simulink model "BLDCctrlBasedOnMBD"  (R2020b)
settings: Solver=FixedStepDiscrete  StartTime=0.0  StopTime=10.0  FixedStep=0.0001  RelTol=1e-3
PreLoadFcn:
  | load('structMotorCtrl.mat');
  | load('structMBDMotorCrtl.mat');
InitFcn:
  | mbd_s32k_consistency_checks(bdroot(gcs));
undefined symbols (not defined in the file or in its folder): External, LQFP, One, Shot, TRGMUX_PDB_TRIG
libraries: mbd_s32k1xx_ec_toolbox x28, mbd_msd_ec_toolbox x2
settings Model: Creator=k  LastModifiedBy=k
settings DataIOCC: ExternalInput=off  InitialState=off  SaveOutput=off  SignalLogging=off  SaveTime=off
settings OptimizationCC: DefaultParameterBehavior=Inlined  EnhancedBackFolding=on  PassReuseOutputArgsAs=Individual arguments  ZeroExternalMemoryAtStartup=off  ZeroInternalMemoryAtStartup=off  OptimizeBlockOrder=speed  DifferentSizesBufferReuse=on  OptimizationCustomize=off  EfficientTunableParamExpr=on
settings DebuggingCC: InheritedTsInSrcMsg=none  SingleTaskRateTransMsg=error  ParameterTunabilityLossMsg=error  UnconnectedInputMsg=error  UnconnectedOutputMsg=error  UnconnectedLineMsg=error  UnknownTsInhSupMsg=error
settings HardwareCC: ProdBitPerPointer=32  ProdBitPerSizeT=32  ProdBitPerPtrDiffT=32  ProdLargestAtomicInteger=Long  ProdLargestAtomicFloat=Double  ProdWordSize=32  ProdHWDeviceType=ARM Compatible->ARM Cortex
settings ModelReferenceCC: ModelReferenceNumInstancesAllowed=Single
settings SFSimCC: MATLABDynamicMemAlloc=off
settings RTWCC: Description=Model Based Design Toolbox S32K1xx Code Generation Target  SystemTargetFile=mbd_s32k.tlc  MakeCommand=mbd_s32k_make_rtw COPY_MDLREF_INCLUDES=0  TemplateMakefile=mbd_s32k.tmf  GenerateReport=on
settings CodeAppCC: ForceParamTrailComments=on  IgnoreCustomStorageClasses=off  OperatorAnnotations=on  SimulinkDataObjDesc=on  SFDataObjDesc=on  InsertBlockDesc=on
settings STFCustomTargetCC: TargetLangStandard=C99 (ISO)  MultiwordLength=256  ConcurrentExecutionCompliant=off  CombineOutputUpdateFcns=on  ERTCustomFileBanners=on  SupportContinuousTime=off  SupportNonInlinedSFcns=off  RemoveResetFunc=on  MATLABClassNameForMDSCustomization=Simulink.SoftwareTarget.ERTCustomization  CPPClassGenCompliant=off  GRTInterface=off  SystemTargetFile=mbd_s32k.tlc
settings ERTTargetCC: TargetLangStandard=C99 (ISO)  ParMdlRefBuildCompliant=off  CompOptLevelCompliant=off  ConcurrentExecutionCompliant=off  ModelStepFunctionPrototypeControlCompliant=off  CPPClassGenCompliant=off  UseToolchainInfoCompliant=off  InlinedParameterPlacement=NonHierarchical  ERTSrcFileBannerTemplate=mbd_ert_code_template.cgt  ERTHdrFileBannerTemplate=mbd_ert_code_template.cgt  ERTDataSrcFileTemplate=mbd_ert_code_template.cgt  ERTDataHdrFileTemplate=mbd_ert_code_template.cgt  ERTCustomFileTemplate=example_file_process.tlc

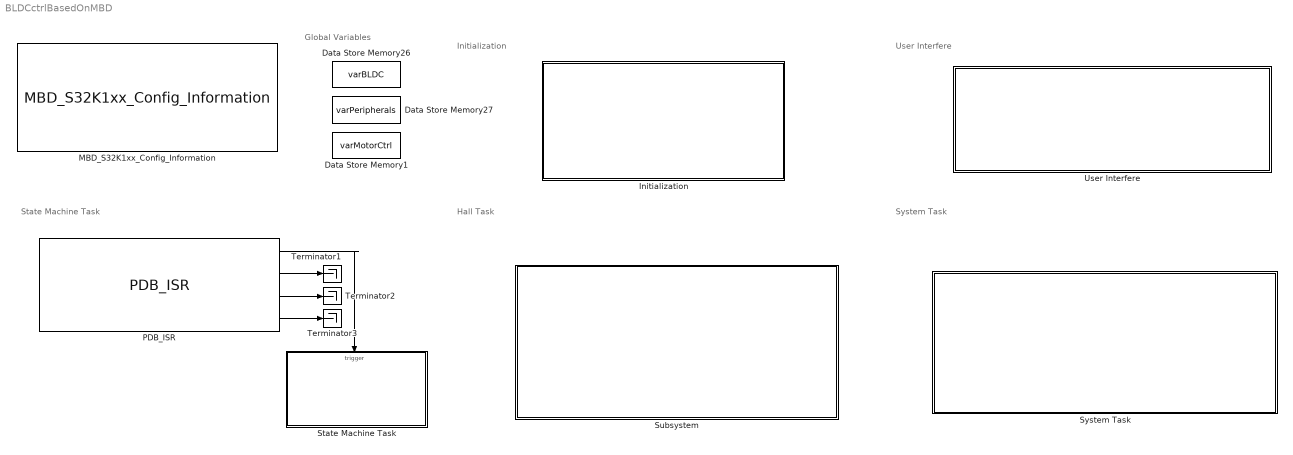
== system BLDCctrlBasedOnMBD ==
  note: State Machine Task
  note: Global Variables
  note: Hall Task
  note: System Task
  note: Initialization
  note: User Interfere
  Data Store Memory1 : DataStoreMemory  DataStoreName=varMotorCtrl  ReadBeforeWriteMsg=warning  WriteAfterWriteMsg=warning  WriteAfterReadMsg=warning  ShowAdditionalParam=off  OutDataTypeStr=Bus: structMotorCtrl
  Data Store Memory26 : DataStoreMemory  DataStoreName=varBLDC  ReadBeforeWriteMsg=warning  WriteAfterWriteMsg=warning  WriteAfterReadMsg=warning  ShowAdditionalParam=off  OutDataTypeStr=Bus: structBLDC
  Data Store Memory27 : DataStoreMemory  DataStoreName=varPeripherals  ReadBeforeWriteMsg=warning  WriteAfterWriteMsg=warning  WriteAfterReadMsg=warning  ShowAdditionalParam=off  OutDataTypeStr=Bus: structPeripherals
  Initialization : Subsystem
  MBD_S32K1xx_Config_Information : mbd_s32k1xx_ec_toolbox/MBD_S32K1xx_Config_Information  mbdt_ver=0  disp_str=|  config_params=[]  mcu_target_name=S32K144  mcu_target_package=100-LQFP  mcu_target_sram_size=64KB  mcu_system_clock_freq=80  mcu_xtal_freq=External 8  mcu_steptick_timer=LPIT Channel 0  mcu_steptick_prio=15  ds_import_enable=on  target_compiler=GCC  target_memory=FLASH  gcc_target_compile_opts=-mthumb -mfloat-abi=hard -mfpu=fpv4-sp-d16 -O1 -g -gstrict-dwarf  gcc_target_assemble_opts=-mthumb -mfloat-abi=hard -mfpu=fpv4-sp-d16 -g  gcc_target_link_opts=-mthumb -mfloat-abi=hard -mfpu=fpv4-sp-d16  gcc_target_default_lcf=on  gcc_target_user_lcf=S32K148_192_flash.ld  ghs_target_compile_opts=-cpu=cortexm4f -thumb -fpu=vfpv4_d16 -fsingle -Ogeneral -Wundef -Wimplicit-int -Wshadow -Wtrigraphs --no_commons --gnu_asm -gnu99 -gdwarf-2 -G  ghs_target_assemble_opts=-cpu=cortexm4f -fpu=vfpv4_d16  ghs_target_link_opts=-cpu=cortexm4f -thumb -fpu=vfpv4_d16  ghs_target_default_lcf=on  ghs_target_user_lcf=S32K148_192_flash.ld  iar_target_compile_opts=--cpu=Cortex-M4F --thumb --fpu=VFPv4_sp -Ol -e --debug --dlib_config normal  iar_target_assemble_opts=--cpu Cortex-M4F --thumb --fpu VFPv4_sp  iar_target_link_opts=--no_exceptions --vfe --inline  iar_target_default_lcf=on  iar_target_user_lcf=S32K148_192_flash.icf  pil_download_enable=off  rbl_download_enable=on  rbl_start_delay=5000  rbl_download_interface=OpenSDA  rbl_restart_request=off  rbl_com_port=Custom  rbl_com_port_custom=COM1  pil_download_rate=57600  pil_opensda_drive=Custom  pil_opensda_drive_custom=E  pil_uart_instance=1  pil_uart_rx=PTC6: [LPUART1_RX | Receive]  pil_uart_tx=PTC7: [LPUART1_TX | Transmit]  FTM_PWM_PcrCheckEnDis=on  FTM_Input_Edge_Inputs_PcrCheckEnDis=on  FTM_Dual_Edge_Inputs_PcrCheckEnDis=on  FTM_Quadrature_Inputs_PcrCheckEnDis=on  FTM_Hall_Sensor_Inputs_PcrCheckEnDis=on  LPTMR_PcrCheckEnDis=on  PIT_PcrCheckEnDis=on  RTC_PcrCheckEnDis=on  FlexCAN_PcrCheckEnDis=on  LIN_PcrCheckEnDis=on  FlexIO_PcrCheckEnDis=on  LPI2C_PcrCheckEnDis=on  LPSPI_PcrCheckEnDis=on  LPUART_PcrCheckEnDis=on  CMP_PcrCheckEnDis=on  GPIO_OutputPcrCheckEnDis=on  GPIO_InputPcrCheckEnDis=on  SBC_PcrCheckEnDis=on  BMS_PcrCheckEnDis=on  AMMCLIB_PcrCheckEnDis=on  FM_PcrCheckEnDis=on  Profile_PcrCheckEnDis=on  ConfigParams_PcrCheckEnDis=on  ModelRef_PcrCheckEnDis=on  PDB0_PcrCheckEnDis=on  CSEc_PcrCheckEnDis=on  eDMA_PcrCheckEnDis=on  FLASH_PcrCheckEnDis=on  ADC_PcrCheckEnDis=on  WDOG_PcrCheckEnDis=on
      | Target : S32K144-64KB_SRAM
      | Package : 100-pin
      | System clock : 80 MHz
      | XTAL clock : External 8 MHz
      | Compiler : IAR
      | Target Type : FLASH
      | Download Code after build : off
      | Step Tick Interrupt Priority : 15
  PDB_ISR : mbd_s32k1xx_ec_toolbox/Motor Control Blocks/PDB Blocks/PDB_ISR  Priority=2  pdbModule=0  prioInterrupt=10  regScPdbie=on  regScPdbeie=off  regIdlyIdly=2000
  State Machine Task : Subsystem
  Subsystem : Subsystem
  System Task : Subsystem
  Terminator1 : Terminator
  Terminator2 : Terminator
  Terminator3 : Terminator
  User Interfere : Subsystem
  wires:
  PDB_ISR/2 -> Terminator1/1
  PDB_ISR/3 -> Terminator2/1
  PDB_ISR/4 -> Terminator3/1
  PDB_ISR/1 -> State Machine Task/Trigger

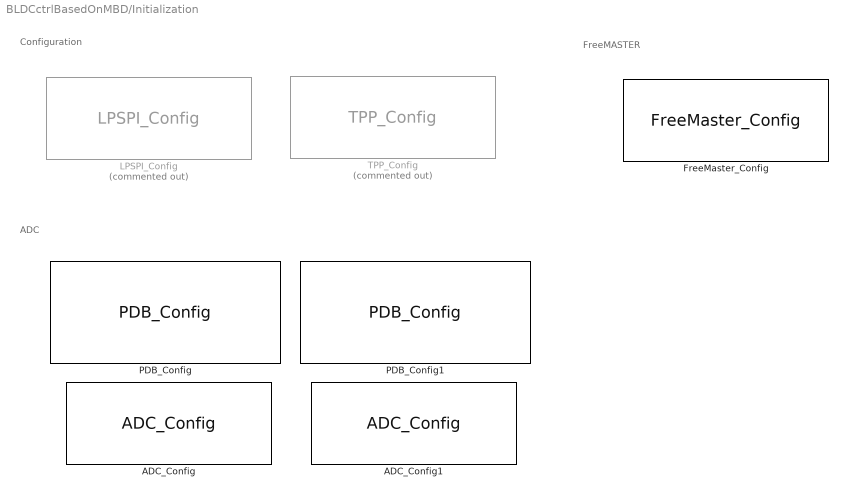
== system BLDCctrlBasedOnMBD/Initialization ==
  note: FreeMASTER
  note: ADC
  note: Configuration
  ADC_Config : mbd_s32k1xx_ec_toolbox/Motor Control Blocks/ADC Blocks/ADC_Config  instance=0  mode=12-bit conversion  smplts=20  adiclk=alternate clock 1  adiv=input clock  show_adv_opts=on  pretrgsel=PDB pre-trigger  swpretrg=Disabled  adtrg=hardware  trgsel=PDB output  refsel=Vrefh and Vrefl  supply_monitoring=off  acfe=off  acfgt=off  acren=off  cv1=0  cv2=0  adco=off  avge=off  avgs=4 samples
  ADC_Config1 : mbd_s32k1xx_ec_toolbox/Motor Control Blocks/ADC Blocks/ADC_Config  instance=1  mode=12-bit conversion  smplts=20  adiclk=alternate clock 1  adiv=input clock  show_adv_opts=on  pretrgsel=PDB pre-trigger  swpretrg=Disabled  adtrg=hardware  trgsel=PDB output  refsel=Vrefh and Vrefl  supply_monitoring=off  acfe=off  acfgt=off  acren=off  cv1=0  cv2=0  adco=off  avge=off  avgs=4 samples
  FreeMaster_Config : mbd_s32k1xx_ec_toolbox/Utility Blocks/FreeMaster_Config  interface=LPUART1  baudrate=115200  rxd=PTC6: [LPUART1_RX | Receive]  txd=PTC7: [LPUART1_TX | Transmit]  mode=Poll-driven  isr_prio=15  show_adv_opts=on  use_scope=on  max_scope_vars=8  use_recorder=on  max_rec_vars=8  rec_buff_size=1024  rec_timebase=0 seconds  comm_buffer_size_auto=on  comm_buffer_size=255  comm_rqueue_size_default=on  comm_rqueue_size=32
  "LPSPI_Config " : mbd_s32k1xx_ec_toolbox/Communication Blocks/SPI Blocks/LPSPI_Config   Commented=on  InstanceNumber=0  Role=Master  BaudRate=2000000  ShowAdvanced=on  sin=PTB3: [LPSPI0_SIN | LPSPI Serial Data Input]  sout=PTB4: [LPSPI0_SOUT | LPSPI Serial Data Output]  sck=PTB2: [LPSPI0_SCK | LPSPI Serial Clock I/O]  pcs0=None  pcs1=None  pcs2=None  pcs3=None  CPHA=1  CPOL=0  BitOrder=MSB first  TransferSize=8  WhichPCS=0  PCSPol=ActiveLow  ContinuousTransfer=off
  PDB_Config : mbd_s32k1xx_ec_toolbox/Motor Control Blocks/PDB Blocks/PDB_Config  pdbModule=0  regScCont=One-Shot  regScTrgsel=External (TRGMUX_PDB_TRIG)  trgMuxSel=FTM3 Initialize Trigger  trgMuxSelPin=PTB5: [TRGMUX_IN0 | Trigger Mux Input]  regModModulus=3900  regScPrescaler=1  regScMult=1  regPoenPoen0=off  regPo0DlyDly1=0  regPo0DlyDly2=0  enable_pdb_init=on  show_adv_opts=on  regCh0C1En0=on  regCh0C1En1=on  regCh0C1En2=on  regCh0C1En3=on  regCh0C1En4=off  regCh0C1En5=off  regCh0C1En6=off  regCh0C1En7=off  regCh0C1Bb0=off  regCh0C1Bb1=off  regCh0C1Bb2=off  regCh0C1Bb3=off  regCh0C1Bb4=off  regCh0C1Bb5=off  regCh0C1Bb6=off  regCh0C1Bb7=off  regCh0C1Tos0=Pre-trigger is in delay mode  regCh0C1Tos1=Pre-trigger is in delay mode  regCh0C1Tos2=Pre-trigger is in delay mode  regCh0C1Tos3=Pre-trigger is in delay mode  regCh0C1Tos4=Pre-trigger is in delay mode  regCh0C1Tos5=Pre-trigger is in delay mode  regCh0C1Tos6=Pre-trigger is in delay mode  regCh0C1Tos7=Pre-trigger is in delay mode  regCh0DlyDly0=0  regCh0DlyDly1=500  regCh0DlyDly2=1000  regCh0DlyDly3=1500  regCh0DlyDly4=0  regCh0DlyDly5=0  regCh0DlyDly6=0  regCh0DlyDly7=0  regCh1C1En0=off  regCh1C1En1=off  regCh1C1En2=off  regCh1C1En3=off  regCh1C1En4=off  regCh1C1En5=off  regCh1C1En6=off  regCh1C1En7=off  regCh1C1Bb0=off  regCh1C1Bb1=off  regCh1C1Bb2=off  regCh1C1Bb3=off  regCh1C1Bb4=off  regCh1C1Bb5=off  regCh1C1Bb6=off  regCh1C1Bb7=off  regCh1C1Tos0=Pre-trigger is in delay mode  regCh1C1Tos1=Pre-trigger is in delay mode  regCh1C1Tos2=Pre-trigger is in delay mode  regCh1C1Tos3=Pre-trigger is in delay mode  regCh1C1Tos4=Pre-trigger is in delay mode  regCh1C1Tos5=Pre-trigger is in delay mode  regCh1C1Tos6=Pre-trigger is in delay mode  regCh1C1Tos7=Pre-trigger is in delay mode  regCh1DlyDly0=0  regCh1DlyDly1=0  regCh1DlyDly2=0  regCh1DlyDly3=0  regCh1DlyDly4=0  regCh1DlyDly5=0  regCh1DlyDly6=0  regCh1DlyDly7=0
  PDB_Config1 : mbd_s32k1xx_ec_toolbox/Motor Control Blocks/PDB Blocks/PDB_Config  pdbModule=1  regScCont=One-Shot  regScTrgsel=External (TRGMUX_PDB_TRIG)  trgMuxSel=FTM3 Initialize Trigger  trgMuxSelPin=PTB5: [TRGMUX_IN0 | Trigger Mux Input]  regModModulus=3900  regScPrescaler=1  regScMult=1  regPoenPoen0=off  regPo0DlyDly1=0  regPo0DlyDly2=0  enable_pdb_init=on  show_adv_opts=on  regCh0C1En0=on  regCh0C1En1=on  regCh0C1En2=off  regCh0C1En3=off  regCh0C1En4=off  regCh0C1En5=off  regCh0C1En6=off  regCh0C1En7=off  regCh0C1Bb0=off  regCh0C1Bb1=off  regCh0C1Bb2=off  regCh0C1Bb3=off  regCh0C1Bb4=off  regCh0C1Bb5=off  regCh0C1Bb6=off  regCh0C1Bb7=off  regCh0C1Tos0=Pre-trigger is in delay mode  regCh0C1Tos1=Pre-trigger is in delay mode  regCh0C1Tos2=Pre-trigger is in delay mode  regCh0C1Tos3=Pre-trigger is in delay mode  regCh0C1Tos4=Pre-trigger is in delay mode  regCh0C1Tos5=Pre-trigger is in delay mode  regCh0C1Tos6=Pre-trigger is in delay mode  regCh0C1Tos7=Pre-trigger is in delay mode  regCh0DlyDly0=0  regCh0DlyDly1=1000  regCh0DlyDly2=0  regCh0DlyDly3=0  regCh0DlyDly4=0  regCh0DlyDly5=0  regCh0DlyDly6=0  regCh0DlyDly7=0  regCh1C1En0=off  regCh1C1En1=off  regCh1C1En2=off  regCh1C1En3=off  regCh1C1En4=off  regCh1C1En5=off  regCh1C1En6=off  regCh1C1En7=off  regCh1C1Bb0=off  regCh1C1Bb1=off  regCh1C1Bb2=off  regCh1C1Bb3=off  regCh1C1Bb4=off  regCh1C1Bb5=off  regCh1C1Bb6=off  regCh1C1Bb7=off  regCh1C1Tos0=Pre-trigger is in delay mode  regCh1C1Tos1=Pre-trigger is in delay mode  regCh1C1Tos2=Pre-trigger is in delay mode  regCh1C1Tos3=Pre-trigger is in delay mode  regCh1C1Tos4=Pre-trigger is in delay mode  regCh1C1Tos5=Pre-trigger is in delay mode  regCh1C1Tos6=Pre-trigger is in delay mode  regCh1C1Tos7=Pre-trigger is in delay mode  regCh1DlyDly0=0  regCh1DlyDly1=0  regCh1DlyDly2=0  regCh1DlyDly3=0  regCh1DlyDly4=0  regCh1DlyDly5=0  regCh1DlyDly6=0  regCh1DlyDly7=0
  TPP_Config : mbd_msd_ec_toolbox/TPP/TPP_Config  Priority=1  Commented=on  tppInstance=0  desatMode=off  fullonMode=on  lockMode=off  overtempEvent=on  phaseEvent=on  desatEvent=on  framingEvent=on  vlsEvent=on  writeErrEvent=on  overcurrentEvent=on  resetEvent=on  mcuTppIntEn=on  prioInt=15  tppDeadtime=500  initTppNow=on  tppSpiInst=Please add SPI block to workspace  tppPwmModule=Please add FTM block to workspace  tppPair0_1=on  tppPair2_3=on  tppPair4_5=on  tppPair6_7=off  tppFirstChHS=on  tppEn1Pin=PTA2: [PTA2 | Port A I/O]  tppEn2Pin=PTA2: [PTA2 | Port A I/O]  tppRstPin=PTA3: [PTA3 | Port A I/O]  tppCsPin=PTB5: [PTB5 | Port B I/O]  tppIntPin=PTE10: [PTE10 | Port E I/O]

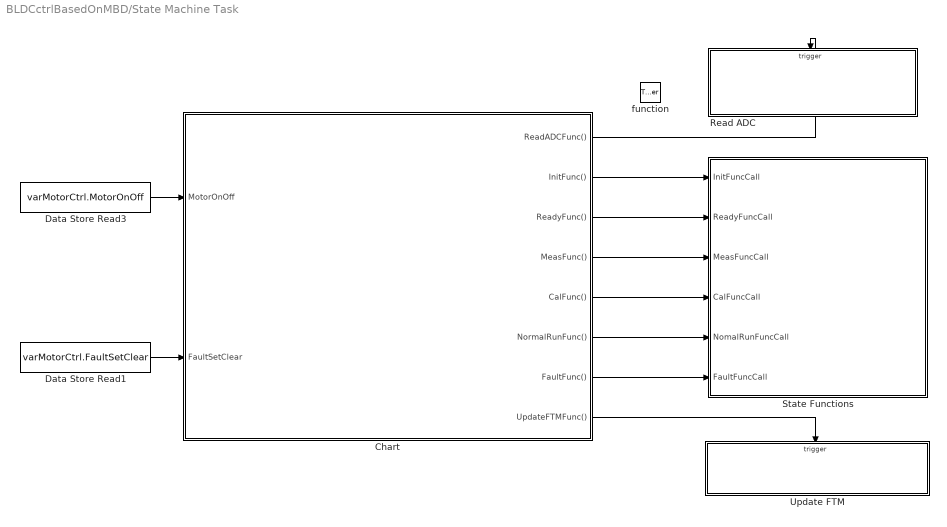
== system BLDCctrlBasedOnMBD/State Machine Task ==
  function : TriggerPort  TriggerType=function-call  VariantControl=Variant
  Chart : Stateflow chart  TreatAsAtomicUnit=on
      settings: PortSchema="{\"entries\":[{\"content\":{\"sides\":[{\"content\":{\"connectorIds\":[\"In1\",\"In2\"]},\"type\":\"ConnectorPlacement.EquallySpacedRectSide\",\"uuid\":\"6aab3670-dbd5-4778-9051-de706f320d6c\"},{\"content\":{\"connectorIds\":[\"Out7\",\"Out2\",\"Out3\",\"Out1\",\"Out4\",\"Out5\",\"Out6\",\"Out8\"],\"side\":\"RIGHT\"},\"type\":\"ConnectorPlacement.EquallySpacedRectSide\",\"uuid\":\"2f9f0170-7a01-4f36-b182-da63b20b6c86\"},{\"content\":{\"connectorIds\":[],\"side\":\"TOP\"},\"type\":\"ConnectorPlacement.EquallySpacedRectSide\",\"uuid\":\"ed2088fa-8282-455e-b501-bc381afe58e4\"},{\"content\":{\"connectorIds\":[],\"side\":\"HIDDEN\"},\"type\":\"ConnectorPlacement.EquallySpacedRectSide\",\"uuid\":\"d652818b-6052-4db5-9e3c-1b8d8b3f5bf8\"}]},\"type\":\"ConnectorPlacement.EquallySpacedConnector\",\"uuid\":\"e57e4f41-1290-4580-a9fc-0c62073a8c32\"}],\"packageUris\":[\"http://schema.mathworks.com/mf0/Connector/R2020b\"],\"version\":\"1.0\"}"
  Data Store Read1 : DataStoreRead  DataStoreName=varMotorCtrl  DataStoreElements=varMotorCtrl.FaultSetClear
  Data Store Read3 : DataStoreRead  DataStoreName=varMotorCtrl  DataStoreElements=varMotorCtrl.MotorOnOff
  Read ADC : Subsystem  TreatAsAtomicUnit=on
  State Functions : Subsystem  Priority=1
  Update FTM : Subsystem
  wires:
  Data Store Read3/1 -> Chart/1(MotorOnOff)
  Data Store Read1/1 -> Chart/2(FaultSetClear)
  Chart/7(ReadADCFunc()) -> Read ADC/Trigger
  Chart/8(UpdateFTMFunc()) -> Update FTM/Trigger
  Chart/2(InitFunc()) -> State Functions/1(InitFuncCall)
  Chart/3(ReadyFunc()) -> State Functions/2(ReadyFuncCall)
  Chart/1(MeasFunc()) -> State Functions/3(MeasFuncCall)
  Chart/4(CalFunc()) -> State Functions/4(CalFuncCall)
  Chart/5(NormalRunFunc()) -> State Functions/5(NomalRunFuncCall)
  Chart/6(FaultFunc()) -> State Functions/6(FaultFuncCall)

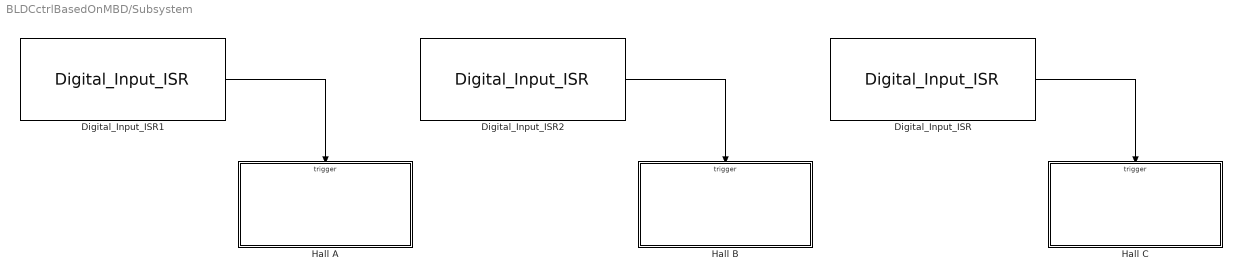
== system BLDCctrlBasedOnMBD/Subsystem ==
  Digital_Input_ISR : mbd_s32k1xx_ec_toolbox/GPIO Blocks/Digital_Input_ISR  gpio_pin=PTA1: [PTA1 | Port A I/O]  irqc=on either-edge  prio=5
  Digital_Input_ISR1 : mbd_s32k1xx_ec_toolbox/GPIO Blocks/Digital_Input_ISR  gpio_pin=PTA15: [PTA15 | Port A I/O]  irqc=on either-edge  prio=5
  Digital_Input_ISR2 : mbd_s32k1xx_ec_toolbox/GPIO Blocks/Digital_Input_ISR  gpio_pin=PTA16: [PTA16 | Port A I/O]  irqc=on either-edge  prio=5
  Hall A : Subsystem  TreatAsAtomicUnit=on
  Hall B : Subsystem  TreatAsAtomicUnit=on
  Hall C : Subsystem  TreatAsAtomicUnit=on
  wires:
  Digital_Input_ISR/1 -> Hall C/Trigger
  Digital_Input_ISR1/1 -> Hall A/Trigger
  Digital_Input_ISR2/1 -> Hall B/Trigger

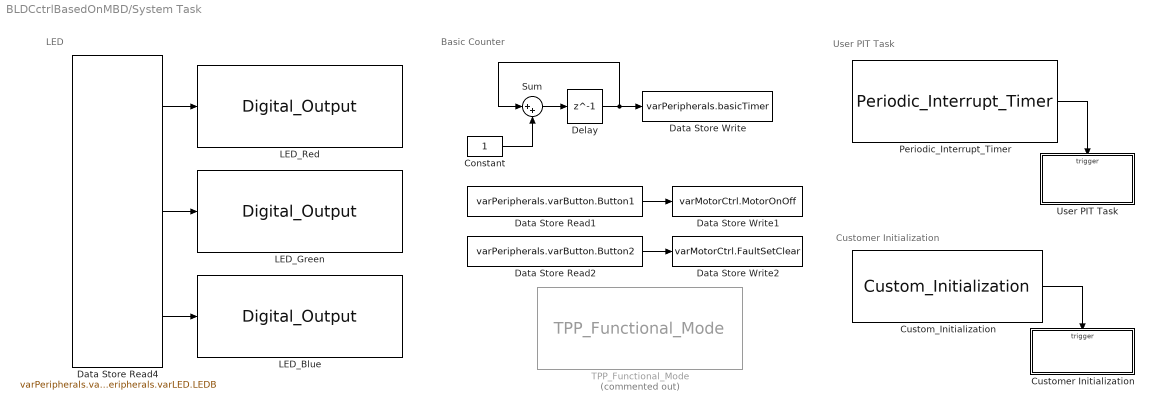
== system BLDCctrlBasedOnMBD/System Task ==
  note: LED
  note: Basic Counter
  note: User PIT Task
  note: Customer Initialization
  Constant : Constant  OutDataTypeStr=uint32
  Custom_Initialization : mbd_s32k1xx_ec_toolbox/Utility Blocks/Custom_Initialization
  Customer Initialization : Subsystem  TreatAsAtomicUnit=on
  Data Store Read1 : DataStoreRead  DataStoreName=varPeripherals  DataStoreElements=varPeripherals.varButton.Button1
  Data Store Read2 : DataStoreRead  DataStoreName=varPeripherals  DataStoreElements=varPeripherals.varButton.Button2
  Data Store Read4 : DataStoreRead  DataStoreName=varPeripherals  DataStoreElements=varPeripherals.varLED.LEDR#varPeripherals.varLED.LEDG#varPeripherals.varLED.LEDB
  Data Store Write : DataStoreWrite  DataStoreName=varPeripherals  DataStoreElements=varPeripherals.basicTimer
  Data Store Write1 : DataStoreWrite  DataStoreName=varMotorCtrl  DataStoreElements=varMotorCtrl.MotorOnOff
  Data Store Write2 : DataStoreWrite  DataStoreName=varMotorCtrl  DataStoreElements=varMotorCtrl.FaultSetClear
  Delay : Delay  DelayLength=1  InitialCondition=0
  LED_Blue : mbd_s32k1xx_ec_toolbox/GPIO Blocks/Digital_Output  gpio_pin=PTD0: [PTD0 | Port D I/O]  init_val=High  drive_strength=Low
  LED_Green : mbd_s32k1xx_ec_toolbox/GPIO Blocks/Digital_Output  gpio_pin=PTD16: [PTD16 | Port D I/O]  init_val=High  drive_strength=Low
  LED_Red : mbd_s32k1xx_ec_toolbox/GPIO Blocks/Digital_Output  gpio_pin=PTD15: [PTD15 | Port D I/O]  init_val=High  drive_strength=Low
  Periodic_Interrupt_Timer : mbd_s32k1xx_ec_toolbox/Utility Blocks/Periodic_Interrupt_Timer  channel=1  period=500000  prio=14  startCounter=on
  Sum : Sum  Inputs=|++
  TPP_Functional_Mode : mbd_msd_ec_toolbox/TPP/TPP_Functional_Mode  Commented=on  tppInstance=0  action=Sleep
  User PIT Task : Subsystem  TreatAsAtomicUnit=on
  wires:
  Data Store Read4/1 -> LED_Red/1
  Data Store Read4/2 -> LED_Green/1
  Data Store Read4/3 -> LED_Blue/1
  Constant/1 -> Sum/2
  Delay/1 -> Data Store Write/1, Sum/1
  Sum/1 -> Delay/1
  Periodic_Interrupt_Timer/1 -> User PIT Task/Trigger
  Custom_Initialization/1 -> Customer Initialization/Trigger
  Data Store Read1/1 -> Data Store Write1/1
  Data Store Read2/1 -> Data Store Write2/1

== system BLDCctrlBasedOnMBD/User Interfere ==
  note: User Button
  Digital_Input_ISR : mbd_s32k1xx_ec_toolbox/GPIO Blocks/Digital_Input_ISR  gpio_pin=PTC12: [PTC12 | Port C I/O]  irqc=on rising-edge  prio=13
  Digital_Input_ISR1 : mbd_s32k1xx_ec_toolbox/GPIO Blocks/Digital_Input_ISR  gpio_pin=PTC13: [PTC13 | Port C I/O]  irqc=on rising-edge  prio=13
  Function-Call Subsystem1 : Subsystem  TreatAsAtomicUnit=on
  Function-Call Subsystem2 : Subsystem  TreatAsAtomicUnit=on
  wires:
  Digital_Input_ISR/1 -> Function-Call Subsystem2/Trigger
  Digital_Input_ISR1/1 -> Function-Call Subsystem1/Trigger

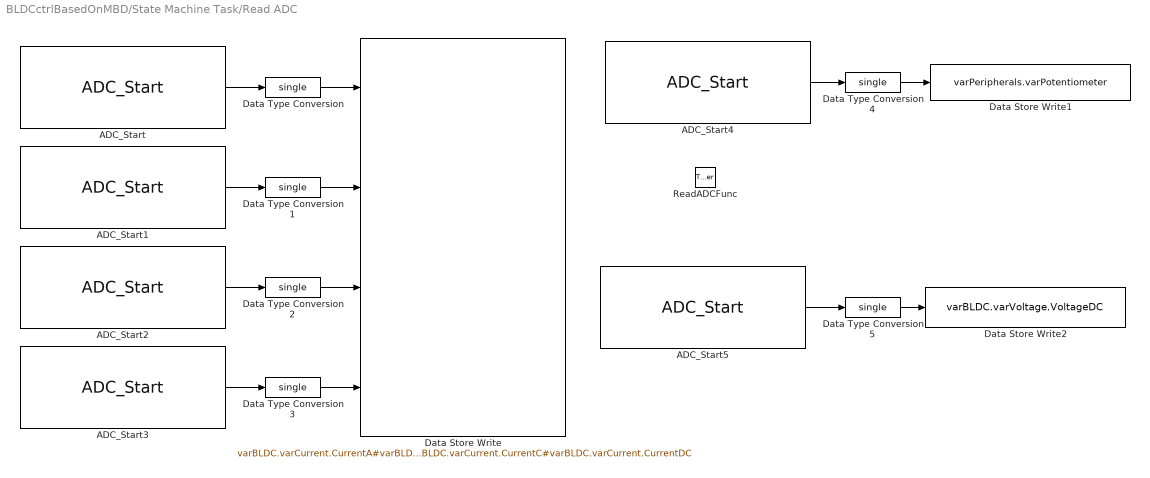
== system BLDCctrlBasedOnMBD/State Machine Task/Read ADC ==
  ReadADCFunc : TriggerPort  TriggerType=function-call  VariantControl=Variant
  ADC_Start : mbd_s32k1xx_ec_toolbox/Motor Control Blocks/ADC Blocks/ADC_Start  instance=0  adc_r=A  adc_chan=VREFSH  aien=off  mcuTargetUpdate=on
  ADC_Start1 : mbd_s32k1xx_ec_toolbox/Motor Control Blocks/ADC Blocks/ADC_Start  instance=0  adc_r=B  adc_chan=VREFSL  aien=off  mcuTargetUpdate=on
  ADC_Start2 : mbd_s32k1xx_ec_toolbox/Motor Control Blocks/ADC Blocks/ADC_Start  instance=0  adc_r=C  adc_chan=VDD 3V  aien=off  mcuTargetUpdate=on
  ADC_Start3 : mbd_s32k1xx_ec_toolbox/Motor Control Blocks/ADC Blocks/ADC_Start  instance=0  adc_r=D  adc_chan=PTC14: [ADC0_SE12 | ADC Single Ended Input]  aien=off  mcuTargetUpdate=on
  ADC_Start4 : mbd_s32k1xx_ec_toolbox/Motor Control Blocks/ADC Blocks/ADC_Start  instance=1  adc_r=A  adc_chan=VREFSH  aien=off  mcuTargetUpdate=on
  ADC_Start5 : mbd_s32k1xx_ec_toolbox/Motor Control Blocks/ADC Blocks/ADC_Start  instance=1  adc_r=B  adc_chan=VREFSL  aien=off  mcuTargetUpdate=on
  Data Store Write : DataStoreWrite  DataStoreName=varBLDC  DataStoreElements=varBLDC.varCurrent.CurrentA#varBLDC.varCurrent.CurrentB#varBLDC.varCurrent.CurrentC#varBLDC.varCurrent.CurrentDC
  Data Store Write1 : DataStoreWrite  DataStoreName=varPeripherals  DataStoreElements=varPeripherals.varPotentiometer
  Data Store Write2 : DataStoreWrite  DataStoreName=varBLDC  DataStoreElements=varBLDC.varVoltage.VoltageDC
  Data Type Conversion{,1..5} (6 alike) : DataTypeConversion  OutDataTypeStr=single
  wires:
  ADC_Start/1 -> Data Type Conversion/1
  ADC_Start1/1 -> Data Type Conversion1/1
  ADC_Start2/1 -> Data Type Conversion2/1
  ADC_Start3/1 -> Data Type Conversion3/1
  ADC_Start4/1 -> Data Type Conversion4/1
  ADC_Start5/1 -> Data Type Conversion5/1
  Data Type Conversion/1 -> Data Store Write/1
  Data Type Conversion1/1 -> Data Store Write/2
  Data Type Conversion2/1 -> Data Store Write/3
  Data Type Conversion3/1 -> Data Store Write/4
  Data Type Conversion4/1 -> Data Store Write1/1
  Data Type Conversion5/1 -> Data Store Write2/1

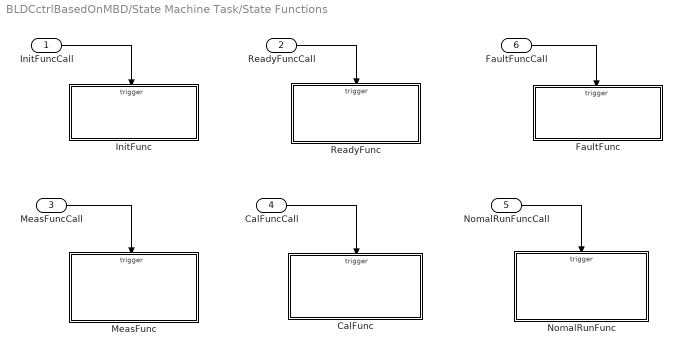
== system BLDCctrlBasedOnMBD/State Machine Task/State Functions ==
  InitFuncCall : Inport
  ReadyFuncCall : Inport  Port=2
  MeasFuncCall : Inport  Port=3
  CalFuncCall : Inport  Port=4
  NomalRunFuncCall : Inport  Port=5
  FaultFuncCall : Inport  Port=6
  CalFunc : Subsystem  TreatAsAtomicUnit=on
  FaultFunc : Subsystem  TreatAsAtomicUnit=on
  InitFunc : Subsystem  TreatAsAtomicUnit=on
  MeasFunc : Subsystem  TreatAsAtomicUnit=on
  NomalRunFunc : Subsystem  TreatAsAtomicUnit=on
  ReadyFunc : Subsystem  TreatAsAtomicUnit=on
  wires:
  MeasFuncCall/1 -> MeasFunc/Trigger
  CalFuncCall/1 -> CalFunc/Trigger
  InitFuncCall/1 -> InitFunc/Trigger
  ReadyFuncCall/1 -> ReadyFunc/Trigger
  FaultFuncCall/1 -> FaultFunc/Trigger
  NomalRunFuncCall/1 -> NomalRunFunc/Trigger

== system BLDCctrlBasedOnMBD/State Machine Task/Update FTM ==
  UpdateFTMFunc : TriggerPort  TriggerType=function-call  VariantControl=Variant
  Data Store Read2 : DataStoreRead  DataStoreName=varBLDC  DataStoreElements=varBLDC.varDuty.DutyA#varBLDC.varDuty.DutyB#varBLDC.varDuty.DutyC
  FTM_PWM_Config : mbd_s32k1xx_ec_toolbox/Motor Control Blocks/FTM Blocks/FTM_PWM_Config  Priority=5  ftmModule=3  ftmMode=Center-Aligned PWM  ftmSourceClock=80 MHz  swcontrol_enable=off  chan0En=on  chan0Type=Independent  chan2En=on  chan2Type=Independent  chan4En=on  chan4Type=Independent  chan6En=off  chan6Type=Independent  ftmPwmUnits=Hz  outFrequency=20000  ftmPeriod=4000  ftmPrescaler=Divide by 1  deadtimeUnits=Nanoseconds  deadtimeNs=0  deadtimeTicks=0  deadtimePrescaler=Divide by 1  dutyCycleCh0=0  dutyCycleCh1=0  dutyCycleCh2=0  dutyCycleCh3=0  dutyCycleCh4=0  dutyCycleCh5=0  dutyCycleCh6=0.25  dutyCycleCh7=0.25  dutyCycleSim=off  startAfterInit=on  showAdvOpt=on  pinFtmCh0=PTB8: [FTM3_CH0 | FTM Channel]  pinFtmCh1=PTB9: [FTM3_CH1 | FTM Channel]  pinPolCh0=Active Low  pinPolCh1=Active High  outputComplem0=Main duplicated  outputLevel0=Low  outputLevel1=Low  pinFtmCh2=PTB10: [FTM3_CH2 | FTM Channel]  pinFtmCh3=PTB11: [FTM3_CH3 | FTM Channel]  pinPolCh2=Active Low  pinPolCh3=Active High  outputComplem2=Main duplicated  outputLevel2=Low  outputLevel3=Low  pinFtmCh4=PTC10: [FTM3_CH4 | FTM Channel]  pinFtmCh5=PTC11: [FTM3_CH5 | FTM Channel]  pinPolCh4=Active Low  pinPolCh5=Active High  outputComplem4=Main duplicated  outputLevel4=Low  outputLevel5=Low  pinFtmCh6=PTC12: [FTM3_CH6 | FTM Channel]  pinFtmCh7=None  pinPolCh6=Active Low  pinPolCh7=Active Low  outputComplem6=Main duplicated  outputLevel6=Low  outputLevel7=Low  initTrigger=on  chTrigger0=off  chTrigger1=off  chTrigger2=off  chTrigger3=off  chTrigger4=off  chTrigger5=off  chTrigger6=off  chTrigger7=off  mcuTargetUpdate=on  pwmSyncTrg=Software trigger  pwmSyncHwRouting=TRGMUX_FTM7  pwmSyncTrg0=off  pwmSyncTrg1=off  pwmSyncTrg2=off  pwmSyncAutoClear=off  pwmSyncMinLoad=on  pwmSyncMaxLoad=off  pwmSyncInvert=PWM Syncronization  pwmSyncOutControl=PWM Syncronization  pwmSyncOutMask=PWM Syncronization  pwmSyncCounterInitial=PWM Syncronization  pwmSyncPoints=Wait Loading Points  reloadEnable=off  reloadPriority=15  reloadHalfCycle=off  reloadHCR=0  reloadFrequency=0  chnMatch0=off  chnMatch1=off  chnMatch2=off  chnMatch3=off  chnMatch4=off  chnMatch5=off  chnMatch6=off  chnMatch7=off  pwmFaultProtection=off  pwmFaultInterrupt=off  pwmFaultClearing=Fault control disabled  pwmFaultPinState=Safe Value  pwmFaultFilterValue=0  pwmFaultPriority=15  fault_disen_0=off  fault_filter_0=off  fault_polarity_0=Active High  fault_disen_1=off  fault_filter_1=off  fault_polarity_1=Active high  fault_disen_2=off  fault_filter_2=off  fault_polarity_2=Active high  fault_disen_3=off  fault_filter_3=off  fault_polarity_3=Active high  fault_pin_0=None  fault_pin_1=None  fault_pin_2=None  fault_pin_3=None
  wires:
  Data Store Read2/1 -> FTM_PWM_Config/1, FTM_PWM_Config/2
  Data Store Read2/3 -> FTM_PWM_Config/5, FTM_PWM_Config/6
  Data Store Read2/2 -> FTM_PWM_Config/3, FTM_PWM_Config/4

== system BLDCctrlBasedOnMBD/Subsystem/Hall A ==
  ReadHallA : TriggerPort  TriggerType=function-call  VariantControl=Variant
  Data Store Write1 : DataStoreWrite  DataStoreName=varBLDC  DataStoreElements=varBLDC.varHall.HallA
  Digital_Input_HALL_A : mbd_s32k1xx_ec_toolbox/GPIO Blocks/Digital_Input  gpio_pin=PTA15: [PTA15 | Port A I/O]  pull_resistor=None  passive_filter=off
  wires:
  Digital_Input_HALL_A/1 -> Data Store Write1/1

== system BLDCctrlBasedOnMBD/Subsystem/Hall B ==
  ReadHallA : TriggerPort  TriggerType=function-call  VariantControl=Variant
  Data Store Write1 : DataStoreWrite  DataStoreName=varBLDC  DataStoreElements=varBLDC.varHall.HallB
  Digital_Input_HALL_B : mbd_s32k1xx_ec_toolbox/GPIO Blocks/Digital_Input  gpio_pin=PTA16: [PTA16 | Port A I/O]  pull_resistor=None  passive_filter=off
  wires:
  Digital_Input_HALL_B/1 -> Data Store Write1/1

== system BLDCctrlBasedOnMBD/Subsystem/Hall C ==
  ReadHallA : TriggerPort  TriggerType=function-call  VariantControl=Variant
  Data Store Write1 : DataStoreWrite  DataStoreName=varBLDC  DataStoreElements=varBLDC.varHall.HallC
  Digital_Input_HALL_C : mbd_s32k1xx_ec_toolbox/GPIO Blocks/Digital_Input  gpio_pin=PTA1: [PTA1 | Port A I/O]  pull_resistor=None  passive_filter=off
  wires:
  Digital_Input_HALL_C/1 -> Data Store Write1/1

== system BLDCctrlBasedOnMBD/System Task/Customer Initialization ==
  CustInit : TriggerPort  TriggerType=function-call  VariantControl=Variant
  0_uint32 : Constant  Value=0  OutDataTypeStr=uint32
  1_boolean : Constant  OutDataTypeStr=boolean
  Data Store Write : DataStoreWrite  DataStoreName=varPeripherals  DataStoreElements=varPeripherals.varLED.LEDR#varPeripherals.varLED.LEDG#varPeripherals.varLED.LEDB#varPeripherals.basicTimer
  wires:
  1_boolean/1 -> Data Store Write/1, Data Store Write/2, Data Store Write/3
  0_uint32/1 -> Data Store Write/4

== system BLDCctrlBasedOnMBD/System Task/User PIT Task ==
  UserPITFunc : TriggerPort  TriggerType=function-call  VariantControl=Variant

== system BLDCctrlBasedOnMBD/User Interfere/Function-Call Subsystem1 ==
  function : TriggerPort  TriggerType=function-call  VariantControl=Variant
  Data Store Read : DataStoreRead  DataStoreName=varPeripherals  DataStoreElements=varPeripherals.varButton.Button2
  Data Store Write : DataStoreWrite  DataStoreName=varPeripherals  DataStoreElements=varPeripherals.varButton.Button2
  Logical Operator : Logic  Operator=NOT  AllPortsSameDT=off  OutDataTypeStr=boolean
  wires:
  Data Store Read/1 -> Logical Operator/1
  Logical Operator/1 -> Data Store Write/1

== system BLDCctrlBasedOnMBD/User Interfere/Function-Call Subsystem2 ==
  function : TriggerPort  TriggerType=function-call  VariantControl=Variant
  Data Store Read : DataStoreRead  DataStoreName=varPeripherals  DataStoreElements=varPeripherals.varButton.Button1
  Data Store Write : DataStoreWrite  DataStoreName=varPeripherals  DataStoreElements=varPeripherals.varButton.Button1
  Logical Operator : Logic  Operator=NOT  AllPortsSameDT=off  OutDataTypeStr=boolean
  wires:
  Logical Operator/1 -> Data Store Write/1
  Data Store Read/1 -> Logical Operator/1

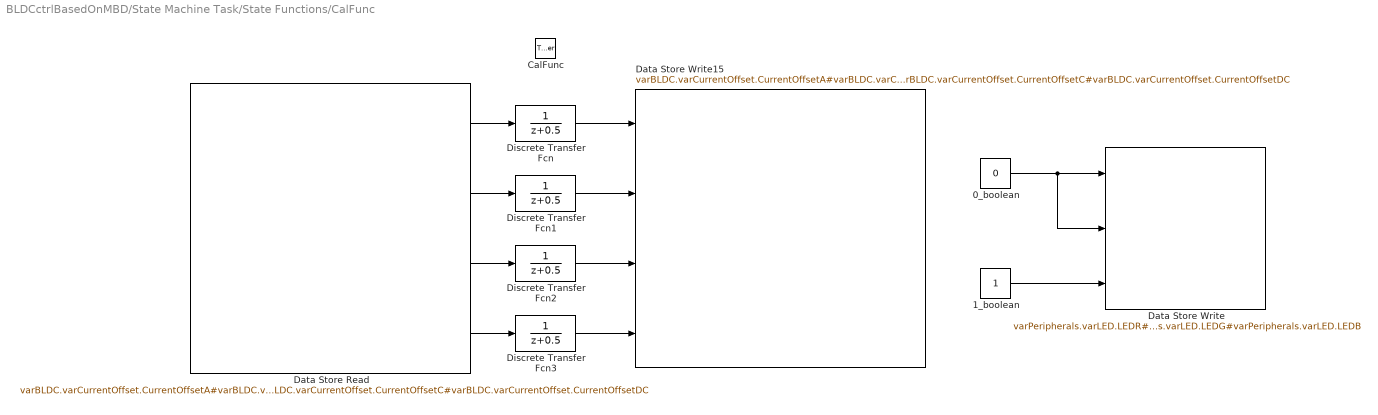
== system BLDCctrlBasedOnMBD/State Machine Task/State Functions/CalFunc ==
  CalFunc : TriggerPort  TriggerType=function-call  VariantControl=Variant
  0_boolean : Constant  Value=0  OutDataTypeStr=boolean
  1_boolean : Constant  OutDataTypeStr=boolean
  Data Store Read : DataStoreRead  DataStoreName=varBLDC  DataStoreElements=varBLDC.varCurrentOffset.CurrentOffsetA#varBLDC.varCurrentOffset.CurrentOffsetB#varBLDC.varCurrentOffset.CurrentOffsetC#varBLDC.varCurrentOffset.CurrentOffsetDC
  Data Store Write : DataStoreWrite  DataStoreName=varPeripherals  DataStoreElements=varPeripherals.varLED.LEDR#varPeripherals.varLED.LEDG#varPeripherals.varLED.LEDB
  Data Store Write15 : DataStoreWrite  DataStoreName=varBLDC  DataStoreElements=varBLDC.varCurrentOffset.CurrentOffsetA#varBLDC.varCurrentOffset.CurrentOffsetB#varBLDC.varCurrentOffset.CurrentOffsetC#varBLDC.varCurrentOffset.CurrentOffsetDC
  Discrete Transfer Fcn{,1..3} (4 alike) : DiscreteTransferFcn
  wires:
  Data Store Read/1 -> Discrete Transfer Fcn/1
  Discrete Transfer Fcn/1 -> Data Store Write15/1
  Data Store Read/2 -> Discrete Transfer Fcn1/1
  Data Store Read/3 -> Discrete Transfer Fcn2/1
  Data Store Read/4 -> Discrete Transfer Fcn3/1
  Discrete Transfer Fcn1/1 -> Data Store Write15/2
  Discrete Transfer Fcn2/1 -> Data Store Write15/3
  Discrete Transfer Fcn3/1 -> Data Store Write15/4
  1_boolean/1 -> Data Store Write/3
  0_boolean/1 -> Data Store Write/2, Data Store Write/1

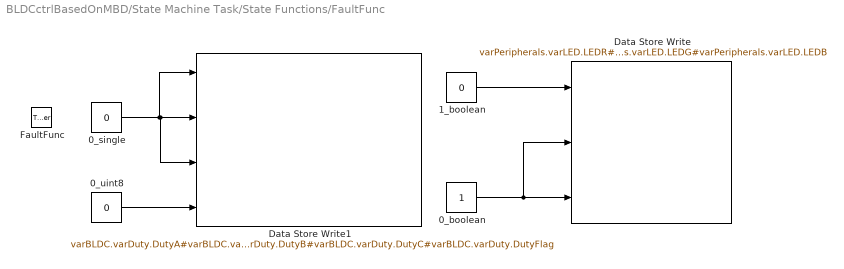
== system BLDCctrlBasedOnMBD/State Machine Task/State Functions/FaultFunc ==
  FaultFunc : TriggerPort  TriggerType=function-call  VariantControl=Variant
  0_boolean : Constant  OutDataTypeStr=boolean
  0_single : Constant  Value=0  OutDataTypeStr=single
  0_uint8 : Constant  Value=0  OutDataTypeStr=uint8
  1_boolean : Constant  Value=0  OutDataTypeStr=boolean
  Data Store Write : DataStoreWrite  DataStoreName=varPeripherals  DataStoreElements=varPeripherals.varLED.LEDR#varPeripherals.varLED.LEDG#varPeripherals.varLED.LEDB
  Data Store Write1 : DataStoreWrite  DataStoreName=varBLDC  DataStoreElements=varBLDC.varDuty.DutyA#varBLDC.varDuty.DutyB#varBLDC.varDuty.DutyC#varBLDC.varDuty.DutyFlag
  wires:
  0_single/1 -> Data Store Write1/3, Data Store Write1/2, Data Store Write1/1
  0_uint8/1 -> Data Store Write1/4
  0_boolean/1 -> Data Store Write/3, Data Store Write/2
  1_boolean/1 -> Data Store Write/1

== system BLDCctrlBasedOnMBD/State Machine Task/State Functions/InitFunc ==
  InitFunc : TriggerPort  TriggerType=function-call  VariantControl=Variant
  0_boolean : Constant  Value=0  OutDataTypeStr=boolean
  0_single : Constant  Value=0  OutDataTypeStr=single
  0_uint8 : Constant  Value=0  OutDataTypeStr=uint8
  Data Store Write5 : DataStoreWrite  DataStoreName=varBLDC  DataStoreElements=varBLDC.varStateFlag.FaultFlag#varBLDC.varStateFlag.InitFlag#varBLDC.varStateFlag.ReadyFlag#varBLDC.varStateFlag.MeasFlag#varBLDC.varStateFlag.CalFlag#varBLDC.varStateFlag.NormalRunFlag#varBLDC.varHall.HallA#varBLDC.varHall.HallB#varBLDC.varHall.HallC#varBLDC.varHallCalc.HallXOR#varBLDC.varHallCalc.HallSum#varBLDC.varHallCalc.HallSpd#varBLDC.varCurrent.CurrentA#varBLDC.varCurrent.CurrentB#varBLDC.varCurrent.CurrentC#varBLDC.varCurrent.CurrentDC#varBLDC.varCurrentOffset.CurrentOffsetA#varBLDC.varCurrentOffset.CurrentOffsetB#varBLDC.varCurrentOffset.CurrentOffsetC#varBLDC.varCurrentOffset.CurrentOffsetDC#varBLDC.varDuty.DutyA#varBLDC.varDuty.DutyB#varBLDC.varDuty.DutyC#varBLDC.varDuty.DutyFlag
  wires:
  0_single/1 -> Data Store Write5/23, Data Store Write5/17, Data Store Write5/16, Data Store Write5/14, Data Store Write5/13, Data Store Write5/12, Data Store Write5/15, Data Store Write5/18, Data Store Write5/19, Data Store Write5/20, Data Store Write5/21, Data Store Write5/22
  0_uint8/1 -> Data Store Write5/11, Data Store Write5/24
  0_boolean/1 -> Data Store Write5/1, Data Store Write5/2, Data Store Write5/5, Data Store Write5/10, Data Store Write5/9, Data Store Write5/8, Data Store Write5/7, Data Store Write5/6, Data Store Write5/4, Data Store Write5/3

== system BLDCctrlBasedOnMBD/State Machine Task/State Functions/MeasFunc ==
  MeasFunc : TriggerPort  TriggerType=function-call  VariantControl=Variant
  Chart : Stateflow chart  TreatAsAtomicUnit=on
  Function-Call Subsystem1 : Subsystem  TreatAsAtomicUnit=on
  Function-Call Subsystem2 : Subsystem  TreatAsAtomicUnit=on
  wires:
  Chart/1(HallDecoder()) -> Function-Call Subsystem1/Trigger
  Chart/2(HallSpdCalc()) -> Function-Call Subsystem2/Trigger

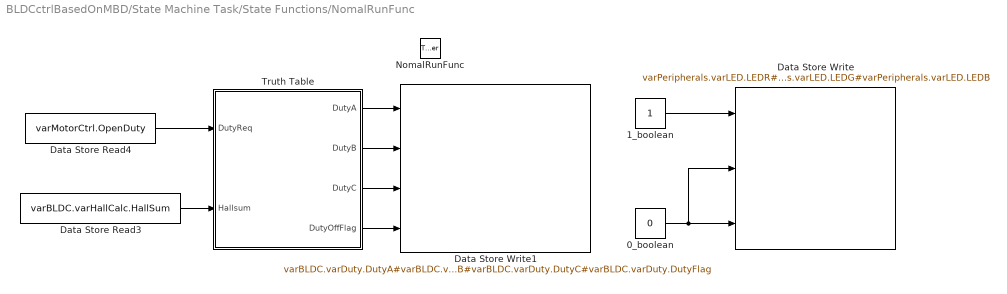
== system BLDCctrlBasedOnMBD/State Machine Task/State Functions/NomalRunFunc ==
  NomalRunFunc : TriggerPort  TriggerType=function-call  VariantControl=Variant
  0_boolean : Constant  Value=0  OutDataTypeStr=boolean
  1_boolean : Constant  OutDataTypeStr=boolean
  Data Store Read3 : DataStoreRead  DataStoreName=varBLDC  DataStoreElements=varBLDC.varHallCalc.HallSum
  Data Store Read4 : DataStoreRead  DataStoreName=varMotorCtrl  DataStoreElements=varMotorCtrl.OpenDuty
  Data Store Write : DataStoreWrite  DataStoreName=varPeripherals  DataStoreElements=varPeripherals.varLED.LEDR#varPeripherals.varLED.LEDG#varPeripherals.varLED.LEDB
  Data Store Write1 : DataStoreWrite  DataStoreName=varBLDC  DataStoreElements=varBLDC.varDuty.DutyA#varBLDC.varDuty.DutyB#varBLDC.varDuty.DutyC#varBLDC.varDuty.DutyFlag
  Truth Table : Truth Table  TreatAsAtomicUnit=on
      settings: PortSchema="{\"entries\":[{\"content\":{\"sides\":[{\"content\":{\"connectorIds\":[\"In2\",\"In1\"]},\"type\":\"ConnectorPlacement.EquallySpacedRectSide\",\"uuid\":\"59c0d94d-4ab6-4082-9c20-9efdae7878b3\"},{\"content\":{\"connectorIds\":[\"Out1\",\"Out2\",\"Out3\",\"Out4\"],\"side\":\"RIGHT\"},\"type\":\"ConnectorPlacement.EquallySpacedRectSide\",\"uuid\":\"fbebaf7f-5920-4df9-84a7-9b0467c91c72\"},{\"content\":{\"connectorIds\":[],\"side\":\"TOP\"},\"type\":\"ConnectorPlacement.EquallySpacedRectSide\",\"uuid\":\"8ff1c87b-d4dc-46a0-9459-25a6278b9f20\"},{\"content\":{\"connectorIds\":[],\"side\":\"HIDDEN\"},\"type\":\"ConnectorPlacement.EquallySpacedRectSide\",\"uuid\":\"16bdd2e1-f1a8-43ed-aa1c-d33053eb9e05\"}]},\"type\":\"ConnectorPlacement.EquallySpacedConnector\",\"uuid\":\"7896656f-e18e-44d5-80e3-9050e65d4579\"}],\"packageUris\":[\"http://schema.mathworks.com/mf0/Connector/R2020b\"],\"version\":\"1.0\"}"
  wires:
  Data Store Read3/1 -> Truth Table/1(Hallsum)
  Truth Table/1(DutyA) -> Data Store Write1/1
  Data Store Read4/1 -> Truth Table/2(DutyReq)
  Truth Table/2(DutyB) -> Data Store Write1/2
  Truth Table/3(DutyC) -> Data Store Write1/3
  Truth Table/4(DutyOffFlag) -> Data Store Write1/4
  0_boolean/1 -> Data Store Write/3, Data Store Write/2
  1_boolean/1 -> Data Store Write/1

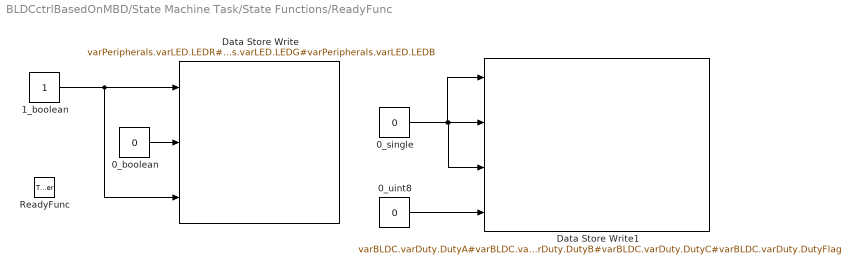
== system BLDCctrlBasedOnMBD/State Machine Task/State Functions/ReadyFunc ==
  ReadyFunc : TriggerPort  TriggerType=function-call  VariantControl=Variant
  0_boolean : Constant  Value=0  OutDataTypeStr=boolean
  0_single : Constant  Value=0  OutDataTypeStr=single
  0_uint8 : Constant  Value=0  OutDataTypeStr=uint8
  1_boolean : Constant  OutDataTypeStr=boolean
  Data Store Write : DataStoreWrite  DataStoreName=varPeripherals  DataStoreElements=varPeripherals.varLED.LEDR#varPeripherals.varLED.LEDG#varPeripherals.varLED.LEDB
  Data Store Write1 : DataStoreWrite  DataStoreName=varBLDC  DataStoreElements=varBLDC.varDuty.DutyA#varBLDC.varDuty.DutyB#varBLDC.varDuty.DutyC#varBLDC.varDuty.DutyFlag
  wires:
  1_boolean/1 -> Data Store Write/3, Data Store Write/1
  0_boolean/1 -> Data Store Write/2
  0_single/1 -> Data Store Write1/3, Data Store Write1/2, Data Store Write1/1
  0_uint8/1 -> Data Store Write1/4

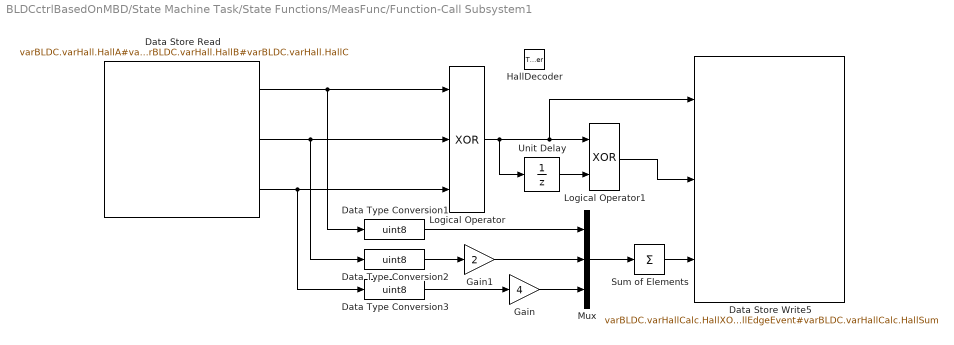
== system BLDCctrlBasedOnMBD/State Machine Task/State Functions/MeasFunc/Function-Call Subsystem1 ==
  HallDecoder : TriggerPort  TriggerType=function-call  VariantControl=Variant
  Data Store Read : DataStoreRead  DataStoreName=varBLDC  DataStoreElements=varBLDC.varHall.HallA#varBLDC.varHall.HallB#varBLDC.varHall.HallC
  Data Store Write5 : DataStoreWrite  DataStoreName=varBLDC  DataStoreElements=varBLDC.varHallCalc.HallXOR#varBLDC.varHallCalc.HallEdgeEvent#varBLDC.varHallCalc.HallSum
  Data Type Conversion1 : DataTypeConversion  OutDataTypeStr=uint8
  Data Type Conversion2 : DataTypeConversion  OutDataTypeStr=uint8
  Data Type Conversion3 : DataTypeConversion  OutDataTypeStr=uint8
  Gain : Gain  Gain=4  OutDataTypeStr=uint8
  Gain1 : Gain  Gain=2  OutDataTypeStr=uint8
  Logical Operator : Logic  Operator=XOR  Inputs=3  AllPortsSameDT=off  OutDataTypeStr=boolean
  Logical Operator1 : Logic  Operator=XOR  AllPortsSameDT=off  OutDataTypeStr=boolean
  Mux : Mux  Inputs=3
  Sum of Elements : Sum  Inputs=+
  Unit Delay : UnitDelay  SampleTime=-1  HasFrameUpgradeWarning=on
  wires:
  Logical Operator/1 -> Data Store Write5/1, Logical Operator1/1, Unit Delay/1
  Unit Delay/1 -> Logical Operator1/2
  Gain/1 -> Mux/3
  Gain1/1 -> Mux/2
  Mux/1 -> Sum of Elements/1
  Sum of Elements/1 -> Data Store Write5/3
  Data Store Read/1 -> Logical Operator/1, Data Type Conversion1/1
  Data Store Read/2 -> Logical Operator/2, Data Type Conversion2/1
  Data Store Read/3 -> Logical Operator/3, Data Type Conversion3/1
  Logical Operator1/1 -> Data Store Write5/2
  Data Type Conversion1/1 -> Mux/1
  Data Type Conversion2/1 -> Gain1/1
  Data Type Conversion3/1 -> Gain/1

== system BLDCctrlBasedOnMBD/State Machine Task/State Functions/MeasFunc/Function-Call Subsystem2 ==
  HallSpdCalc : TriggerPort  TriggerType=function-call  VariantControl=Variant
  Chart : Stateflow chart  TreatAsAtomicUnit=on
  Data Store Read : DataStoreRead  DataStoreName=varBLDC  DataStoreElements=varBLDC.varHallCalc.HallXOR
  Data Store Write1 : DataStoreWrite  DataStoreName=varBLDC  DataStoreElements=varBLDC.varHallCalc.HallSpd
  wires:
  Chart/1(SumOfArray) -> Data Store Write1/1
  Data Store Read/1 -> Chart/1(HallXOR)

== stateflow chart BLDCctrlBasedOnMBD/State Machine Task/State Functions/MeasFunc/Chart ==
  (default) -> (junction 1)
  (junction 1) -> (junction 3) : {HallDecoder;}
  (junction 3) -> (junction 5) : {HallSpdCalc;}
  events: HallDecoder output FUNCTION_CALL_EVENT; HallSpdCalc output FUNCTION_CALL_EVENT

== stateflow chart BLDCctrlBasedOnMBD/State Machine Task/State Functions/MeasFunc/Function-Call Subsystem2/Chart ==
  (default) -> (junction 20)
  (junction 20) -> (junction 1) : [Index > 99]{Index = 0;}
  (junction 1) -> (junction 11) : {RcdArray(Index) = HallXOR;}
  (junction 11) -> (junction 14) : {Index = Index + 1;}
  (junction 14) -> (junction 17) : {SumOfArray = single(sum(RcdArray));}
  data: Index local uint16 =uint16(0); RcdArray local uint8 size=100; SumOfArray output single; HallXOR input boolean

== matlab function BLDCctrlBasedOnMBD/State Machine Task/State Functions/NomalRunFunc/Truth Table ==
  data: Hallsum input uint8; DutyA output single; DutyB output single; DutyC output single; DutyReq input single; DutyOffFlag output uint8
function [DutyA, DutyB, DutyC, DutyOffFlag] = fcn(Hallsum, DutyReq)

aVarTruthTableCondition_1 = false;
aVarTruthTableCondition_2 = false;
aVarTruthTableCondition_3 = false;
aVarTruthTableCondition_4 = false;
aVarTruthTableCondition_5 = false;
aVarTruthTableCondition_6 = false;


% Condition #1
aVarTruthTableCondition_1 = logical(Hallsum == 1);

% Condition #2
aVarTruthTableCondition_2 = logical(Hallsum == 2);

% Condition #3
aVarTruthTableCondition_3 = logical(Hallsum == 3);

% Condition #4
aVarTruthTableCondition_4 = logical(Hallsum == 4);

% Condition #5
aVarTruthTableCondition_5 = logical(Hallsum == 5);

% Condition #6
aVarTruthTableCondition_6 = logical(Hallsum == 6);

if (aVarTruthTableCondition_1 && ~aVarTruthTableCondition_2 && ~aVarTruthTableCondition_3 && ~aVarTruthTableCondition_4 && ~aVarTruthTableCondition_5 && ~aVarTruthTableCondition_6)
    aFcnTruthTableAction_1();
elseif (~aVarTruthTableCondition_1 && aVarTruthTableCondition_2 && ~aVarTruthTableCondition_3 && ~aVarTruthTableCondition_4 && ~aVarTruthTableCondition_5 && ~aVarTruthTableCondition_6)
    aFcnTruthTableAction_2();
elseif (~aVarTruthTableCondition_1 && ~aVarTruthTableCondition_2 && aVarTruthTableCondition_3 && ~aVarTruthTableCondition_4 && ~aVarTruthTableCondition_5 && ~aVarTruthTableCondition_6)
    aFcnTruthTableAction_3();
elseif (~aVarTruthTableCondition_1 && ~aVarTruthTableCondition_2 && ~aVarTruthTableCondition_3 && aVarTruthTableCondition_4 && ~aVarTruthTableCondition_5 && ~aVarTruthTableCondition_6)
    aFcnTruthTableAction_4();
elseif (~aVarTruthTableCondition_1 && ~aVarTruthTableCondition_2 && ~aVarTruthTableCondition_3 && ~aVarTruthTableCondition_4 && aVarTruthTableCondition_5 && ~aVarTruthTableCondition_6)
    aFcnTruthTableAction_5();
elseif (~aVarTruthTableCondition_1 && ~aVarTruthTableCondition_2 && ~aVarTruthTableCondition_3 && ~aVarTruthTableCondition_4 && ~aVarTruthTableCondition_5 && aVarTruthTableCondition_6)
    aFcnTruthTableAction_6();
else % Default
    aFcnTruthTableAction_7();
end

function aFcnTruthTableAction_1()

% Example action 1 called from D1 & D2 column in condition table

DutyA = DutyReq;
DutyB = 0;
DutyC = 0;
DutyOffFlag = 2;

function aFcnTruthTableAction_2()

% Example action 2 called from D3 column in condition table

DutyA = 0;
DutyB = DutyReq;
DutyC = 0;
DutyOffFlag = 3;

function aFcnTruthTableAction_3()



DutyA = 0;
DutyB = DutyReq;
DutyC = 0;
DutyOffFlag = 1;

function aFcnTruthTableAction_4()



DutyA = 0;
DutyB = 0;
DutyC = DutyReq;
DutyOffFlag = 1;

function aFcnTruthTableAction_5()



DutyA = DutyReq;
DutyB = 0;
DutyC = 0;
DutyOffFlag = 3;

function aFcnTruthTableAction_6()



DutyA = 0;
DutyB = 0;
DutyC = DutyReq;
DutyOffFlag = 2;

function aFcnTruthTableAction_7()



DutyA = 0;
DutyB = 0;
DutyC = 0;
DutyOffFlag = 0;

== stateflow chart BLDCctrlBasedOnMBD/State Machine Task/Chart ==
  state ReadADC [parallel]
    ReadADCFunc;
    settings: executionOrder=1
  state StateMachine [parallel]
    settings: executionOrder=2
    state Initial
      en:
      InitFunc;
      InitDone = true;
      bind:InitFunc;
    state Ready
      en:ReadyFunc;
      du:ReadyFunc;
      bind:ReadyFunc;
    state Run
      du:MeasFunc;
      state Calibration
        en:CalCnt = 0;
        du:CalCnt = CalCnt + 1;CalFunc;
        bind:CalFunc;
      state NormalRun
        en:NormalRunFunc;
        du:NormalRunFunc;
        bind:NormalRunFunc;
      (default) -> Calibration
      Calibration -> NormalRun : [CalCnt > 200]
    state Faults
      en:FaultFunc;
      du:FaultFunc;
      bind:FaultFunc;
    (default) -> Initial : {InitDone = false;}
    Initial -> Ready [order 1] : [InitDone]
    Ready -> Run [order 1] : [MotorOnOff]
    Run -> Ready [order 1] : [~MotorOnOff]
    Ready -> Faults [order 2] : [FaultSetClear]
    Faults -> Initial : [~FaultSetClear]
    Initial -> Faults [order 2] : [FaultSetClear]
    Run -> Faults [order 2] : [FaultSetClear]
  state UpdateFTM [parallel]
    UpdateFTMFunc;
    settings: executionOrder=3
  data: CalCnt local; InitDone local boolean; MotorOnOff input boolean; FaultSetClear input boolean
  events: MeasFunc output FUNCTION_CALL_EVENT; InitFunc output FUNCTION_CALL_EVENT; ReadyFunc output FUNCTION_CALL_EVENT; CalFunc output FUNCTION_CALL_EVENT; NormalRunFunc output FUNCTION_CALL_EVENT; FaultFunc output FUNCTION_CALL_EVENT; ReadADCFunc output FUNCTION_CALL_EVENT; UpdateFTMFunc output FUNCTION_CALL_EVENT
